simulink model "FigQ12"  (R2018a)
settings: Solver=VariableStepAuto  StartTime=0.0  StopTime=120  RelTol=1e-3
libraries: slctrlblks x1
settings Model: Creator=Xavier  LastModifiedBy=pt_ptsi

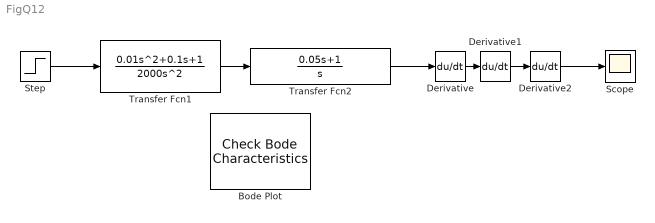
== system FigQ12 ==
  Bode Plot : slctrlblks/Model Verification/Check Bode  Characteristics  InstantiateOnLoad=on  SaveOperatingPoints=off  LinearizationIOs={'/Step', 1, 'in', 'on', '';'/Derivative2', 1, 'out', 'on', ''}  LinearizeAt=SnapshotTimes  SnapshotTimes=[0]  TriggerType=rising  SampleTime=auto  RateConversionMethod=zoh  PreWarpFreq=10  UseExactDelayModel=off  UseFullBlockNameLabels=off  UseBusSignalLabels=off  enabled=on  stopWhenAssertionFail=off  export=off  ViewDlgPos=[100 200 510 390]  OpenViewOnLoad=on  LaunchViewOnOpen=off  FrequencyUnits=rad/s  MagnitudeUnits=dB  PhaseUnits=deg  TimeUnits=seconds  EnableUpperBound=off  UpperBoundFrequencies=[]  UpperBoundMagnitudes=[]  EnableLowerBound=off  LowerBoundFrequencies=[]  LowerBoundMagnitudes=[]
      settings: SourceProductName=Simulink Control Design
  Derivative : Derivative
  Derivative1 : Derivative
  Derivative2 : Derivative
  Scope : Scope
  Step : Step  Time=0  SampleTime=0
  Transfer Fcn1 : TransferFcn  Numerator=[0.01 0.1 1]  Denominator=[2000 0 0]
  Transfer Fcn2 : TransferFcn  Numerator=[0.05 1]  Denominator=[1 0]
  wires:
  Step/1 -> Transfer Fcn1/1
  Transfer Fcn1/1 -> Transfer Fcn2/1
  Transfer Fcn2/1 -> Derivative/1
  Derivative/1 -> Derivative1/1
  Derivative1/1 -> Derivative2/1
  Derivative2/1 -> Scope/1
